simulink subsystem "Transition_Baseline"  (R2024a)
settings: Solver=VariableStepAuto  StartTime=0.0  StopTime=10.0  RelTol=1e-3
undefined symbols (not defined in the file): Kr_transition, Kx_transition, SimIn, SimPar
libraries: simulink_extras x23, ComponentsLib x11, AdaptiveLib x1, libAxisTransformations x1
settings Model: Creator=tbritton  LastModifiedBy=texba
settings SolverCC: AlgebraicLoopSolver=TrustRegion
settings OptimizationCC: ReuseModelBlockBuffer=off
settings DebuggingCC: UnconnectedInputMsg=warning  UnconnectedOutputMsg=warning  UnconnectedLineMsg=warning
settings ModelReferenceCC: EnableRefExpFcnMdlSchedulingChecks=on
settings RTWCC: GPUComputeCapability=3.5  DLArmComputeVersion=19.05

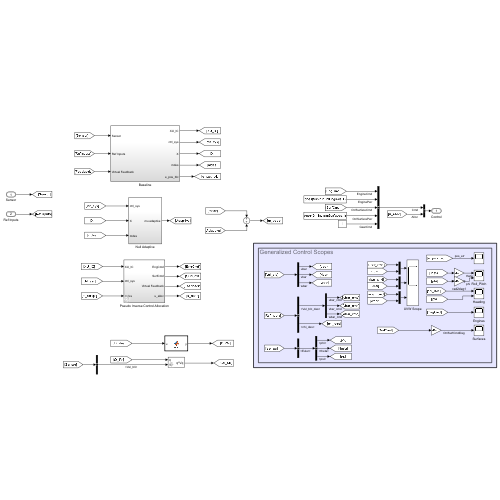
[thumbnail: Simulink's stored preview of the top-level diagram]
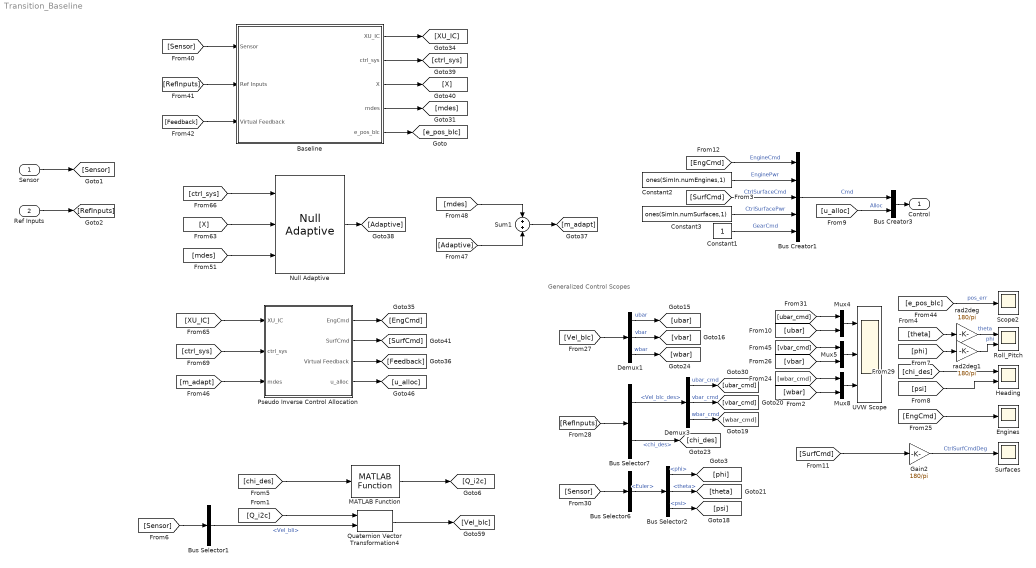
== system Transition_Baseline ==
  note: Generalized Control Scopes
  Sensor : Inport  OutDataTypeStr=Bus: SensorBus
  Ref Inputs : Inport  Port=2  OutDataTypeStr=Bus: BUS_REF_INPUT
  Baseline : Subsystem
      settings: LibrarySourceBlock=ControllersLib/Baseline
  Bus Creator1 : BusCreator  Inputs=5  OutDataTypeStr=Bus: BUS_CMD
  Bus Creator3 : BusCreator  Inputs=2
  Bus Selector1 : BusSelector  OutputSignals=Vel_bIi
  Bus Selector2 : BusSelector  OutputSignals=phi,theta,psi
  Bus Selector6 : BusSelector  OutputSignals=Euler
  Bus Selector7 : BusSelector  OutputSignals=Vel_bIc_des,chi_des
  Constant1 : Constant
  Constant2 : Constant  Value=ones(SimIn.numEngines,1)
  Constant3 : Constant  Value=ones(SimIn.numSurfaces,1)
  Demux1 : Demux  Outputs=3
  Demux3 : Demux  Outputs=3
  Engines : Scope
  Gain2 : Gain  Gain=180/pi
  Heading : Scope  NumInputPorts=2
  MATLAB Function : ComponentsLib/ConvertToControlFrame/MATLAB Function  SystemSampleTime=-1  VariantActivationTime=update diagram  AllowFlexibleInterface=on  Latency=0  AutoFrameSizeCalculation=off
      settings: SourceProductName=Components
  Mux4 : Mux  Inputs=2
  Mux5 : Mux  Inputs=2
  Mux8 : Mux  Inputs=2
  Null Adaptive : AdaptiveLib/Null Adaptive  SystemSampleTime=-1  VariantActivationTime=update diagram  AllowFlexibleInterface=on  Latency=0  AutoFrameSizeCalculation=off
      settings: SourceProductName=Adaptive Augmentation
  Pseudo Inverse Control Allocation : Subsystem  AncestorBlock=AllocatorsLib/Pseudo Inverse Control Allocation
      settings: LibrarySourceBlock=AllocatorsLib/Pseudo Inverse Control Allocation
  Quaternion Vector Transformation4 : libAxisTransformations/Quaternion Vector Transformation  n=0
  Roll_Pitch : Scope  NumInputPorts=2
  Scope2 : Scope
  Sum1 : Sum
  Surfaces : Scope
  UVW Scope : Scope  NumInputPorts=3
  rad2deg : Gain  Gain=180/pi
  rad2deg1 : Gain  Gain=180/pi
  Control : Outport  OutDataTypeStr=Bus: BUS_CONTROL  VectorParamsAs1DForOutWhenUnconnected=off
  wires:
  Baseline/5(e_pos_blc) -> [e_pos_bIc]
  Demux1/1 -> [ubar]  "ubar"
  Mux4/1 -> UVW Scope/1
  Demux3/3 -> [wbar_cmd]  "wbar_cmd"
  Mux5/1 -> UVW Scope/2
  [vbar_cmd] -> Mux5/1
  [ubar_cmd] -> Mux4/1
  [vbar] -> Mux5/2
  [SurfCmd] -> Gain2/1
  [chi_des] -> Heading/1
  [ubar] -> Mux4/2
  [Sensor] -> Bus Selector6/1
  [RefInputs] -> Bus Selector7/1
  [wbar] -> Mux8/2
  [phi] -> rad2deg1/1
  Demux3/2 -> [vbar_cmd]  "vbar_cmd"
  [e_pos_bIc] -> Scope2/1  "pos_err"
  Bus Selector6/1 -> Bus Selector2/1  "<Euler>"
  Bus Selector2/1 -> [phi]  "<phi>"
  Mux8/1 -> UVW Scope/3
  Bus Selector2/3 -> [psi]  "<psi>"
  Gain2/1 -> Surfaces/1  "CtrlSurfCmdDeg"
  [theta] -> rad2deg/1
  Bus Selector2/2 -> [theta]  "<theta>"
  [psi] -> Heading/2
  Demux1/2 -> [vbar]  "vbar"
  [EngCmd] -> Engines/1
  Bus Selector7/1 -> Demux3/1  "<Vel_bIc_des>"
  Demux3/1 -> [ubar_cmd]  "ubar_cmd"
  [Vel_bIc] -> Demux1/1
  Bus Selector7/2 -> [chi_des]  "<chi_des>"
  [wbar_cmd] -> Mux8/1
  Demux1/3 -> [wbar]  "wbar"
  [Sensor] -> Bus Selector1/1
  MATLAB Function/1 -> [Q_i2c]
  Quaternion Vector Transformation4/1 -> [Vel_bIc]
  [chi_des] -> MATLAB Function/1
  [Q_i2c] -> Quaternion Vector Transformation4/1
  Bus Selector1/1 -> Quaternion Vector Transformation4/2  "<Vel_bIi>"
  [ctrl_sys] -> Pseudo Inverse Control Allocation/2(ctrl_sys)
  [XU_IC] -> Pseudo Inverse Control Allocation/1(XU_IC)
  Pseudo Inverse Control Allocation/4(u_alloc) -> [u_alloc]
  Pseudo Inverse Control Allocation/2(SurfCmd) -> [SurfCmd]
  [Adaptive] -> Sum1/2
  [mdes] -> Sum1/1
  Sum1/1 -> [m_adapt]
  Baseline/3(X) -> [X]
  Baseline/2(ctrl_sys) -> [ctrl_sys]
  Null Adaptive/1 -> [Adaptive]
  [X] -> Null Adaptive/2
  [mdes] -> Null Adaptive/3
  [ctrl_sys] -> Null Adaptive/1
  Pseudo Inverse Control Allocation/1(EngCmd) -> [EngCmd]
  Baseline/1(XU_IC) -> [XU_IC]
  Pseudo Inverse Control Allocation/3(Virtual Feedback) -> [Feedback]
  [m_adapt] -> Pseudo Inverse Control Allocation/3(mdes)
  Baseline/4(mdes) -> [mdes]
  [Feedback] -> Baseline/3(Virtual Feedback)
  [RefInputs] -> Baseline/2(Ref Inputs)
  [Sensor] -> Baseline/1(Sensor)
  Constant3/1 -> Bus Creator1/4  "CtrlSurfacePwr"
  Constant2/1 -> Bus Creator1/2  "EnginePwr"
  [EngCmd] -> Bus Creator1/1  "EngineCmd"
  Sensor/1 -> [Sensor]
  Bus Creator1/1 -> Bus Creator3/1  "Cmd"
  [SurfCmd] -> Bus Creator1/3  "CtrlSurfaceCmd"
  Constant1/1 -> Bus Creator1/5  "GearCmd"
  Bus Creator3/1 -> Control/1
  [u_alloc] -> Bus Creator3/2  "Alloc"
  Ref Inputs/1 -> [RefInputs]
  rad2deg/1 -> Roll_Pitch/1  "theta"
  rad2deg1/1 -> Roll_Pitch/2  "phi"

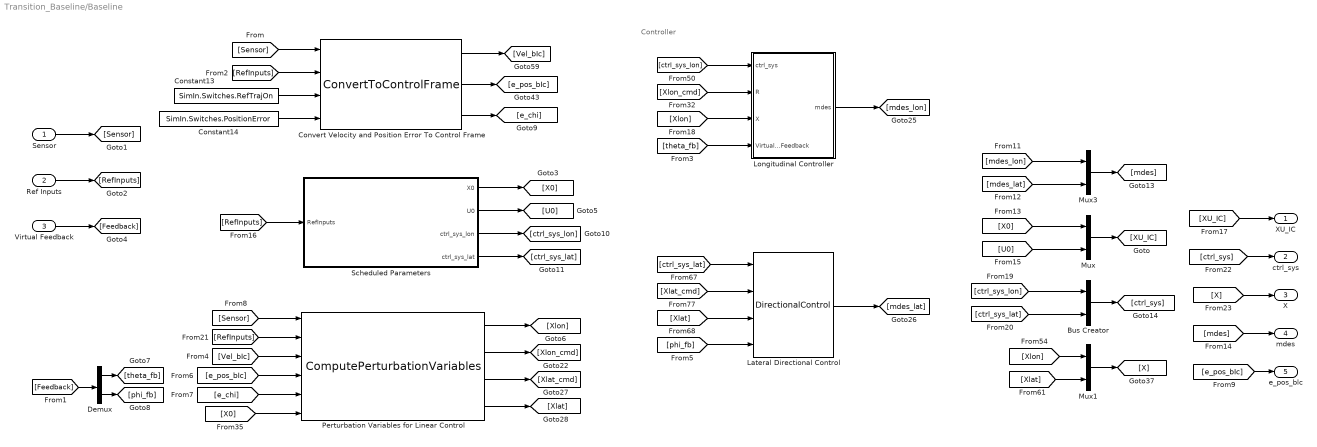
== system Transition_Baseline/Baseline ==
  note: Controller
  Sensor : Inport  OutDataTypeStr=Bus: SensorBus
  Ref Inputs : Inport  Port=2  OutDataTypeStr=Bus: BUS_REF_INPUT
  Virtual Feedback : Inport  Port=3
  Bus Creator : BusCreator  Inputs=2
  Constant13 : Constant  Value=SimIn.Switches.RefTrajOn
  Constant14 : Constant  Value=SimIn.Switches.PositionError
  Convert Velocity and Position Error To Control Frame : ComponentsLib/ConvertToControlFrame  SystemSampleTime=-1  VariantActivationTime=update diagram  AllowFlexibleInterface=on  Latency=0  AutoFrameSizeCalculation=off
      link override delta_cos: Inputs=|++
      settings: SourceProductName=Components
  Demux : Demux  Outputs=2
  Lateral Directional Control : ComponentsLib/DirectionalControl  SystemSampleTime=-1  VariantActivationTime=update diagram  AllowFlexibleInterface=on  Latency=0  AutoFrameSizeCalculation=off
      settings: SourceProductName=Components
  Longitudinal Controller : Subsystem
  Mux : Mux  Inputs=2
  Mux1 : Mux  Inputs=2
  Mux3 : Mux  Inputs=2
  Perturbation Variables for Linear Control : ComponentsLib/ComputePerturbationVariables  SystemSampleTime=-1  VariantActivationTime=update diagram  AllowFlexibleInterface=on  Latency=0  AutoFrameSizeCalculation=off
      settings: SourceProductName=Components
  Scheduled Parameters : Subsystem  AncestorBlock=ComponentsLib/FeedbackScheduling
      settings: LibrarySourceBlock=ComponentsLib/FeedbackScheduling
  XU_IC : Outport
  ctrl_sys : Outport  Port=2
  X : Outport  Port=3
  mdes : Outport  Port=4
  e_pos_blc : Outport  Port=5
  wires:
  [X] -> X/1
  [Xlat] -> Mux1/2
  [Xlon] -> Mux1/1
  Mux1/1 -> [X]
  [ctrl_sys] -> ctrl_sys/1
  Bus Creator/1 -> [ctrl_sys]
  [ctrl_sys_lat] -> Bus Creator/2
  [ctrl_sys_lon] -> Bus Creator/1
  [XU_IC] -> XU_IC/1
  Mux/1 -> [XU_IC]
  [U0] -> Mux/2
  [X0] -> Mux/1
  [mdes] -> mdes/1
  Mux3/1 -> [mdes]
  [mdes_lon] -> Mux3/1
  [phi_fb] -> Lateral Directional Control/4
  [theta_fb] -> Longitudinal Controller/4(Virtual Feedback)
  Demux/1 -> [theta_fb]
  Demux/2 -> [phi_fb]
  [Feedback] -> Demux/1
  Virtual Feedback/1 -> [Feedback]
  [Xlat_cmd] -> Lateral Directional Control/2
  [Xlon] -> Longitudinal Controller/3(X)
  [Xlat] -> Lateral Directional Control/3
  Longitudinal Controller/1(mdes) -> [mdes_lon]
  [ctrl_sys_lon] -> Longitudinal Controller/1(ctrl_sys)
  [ctrl_sys_lat] -> Lateral Directional Control/1
  Lateral Directional Control/1 -> [mdes_lat]
  [Xlon_cmd] -> Longitudinal Controller/2(R)
  Scheduled Parameters/4(ctrl_sys_lat) -> [ctrl_sys_lat]
  Scheduled Parameters/2(U0) -> [U0]
  [e_chi] -> Perturbation Variables for Linear Control/5
  Constant14/1 -> Convert Velocity and Position Error To Control Frame/4
  [RefInputs] -> Perturbation Variables for Linear Control/2
  Constant13/1 -> Convert Velocity and Position Error To Control Frame/3
  [Vel_bIc] -> Perturbation Variables for Linear Control/3
  [Sensor] -> Convert Velocity and Position Error To Control Frame/1
  Convert Velocity and Position Error To Control Frame/3 -> [e_chi]
  Perturbation Variables for Linear Control/2 -> [Xlon_cmd]
  [RefInputs] -> Scheduled Parameters/1(RefInputs)
  Perturbation Variables for Linear Control/4 -> [Xlat]
  [e_pos_bIc] -> Perturbation Variables for Linear Control/4
  Scheduled Parameters/3(ctrl_sys_lon) -> [ctrl_sys_lon]
  Convert Velocity and Position Error To Control Frame/2 -> [e_pos_bIc]
  Convert Velocity and Position Error To Control Frame/1 -> [Vel_bIc]
  [RefInputs] -> Convert Velocity and Position Error To Control Frame/2
  Ref Inputs/1 -> [RefInputs]
  Scheduled Parameters/1(X0) -> [X0]
  Sensor/1 -> [Sensor]
  Perturbation Variables for Linear Control/3 -> [Xlat_cmd]
  [Sensor] -> Perturbation Variables for Linear Control/1
  Perturbation Variables for Linear Control/1 -> [Xlon]
  [X0] -> Perturbation Variables for Linear Control/6
  [e_pos_bIc] -> e_pos_blc/1
  [mdes_lat] -> Mux3/2

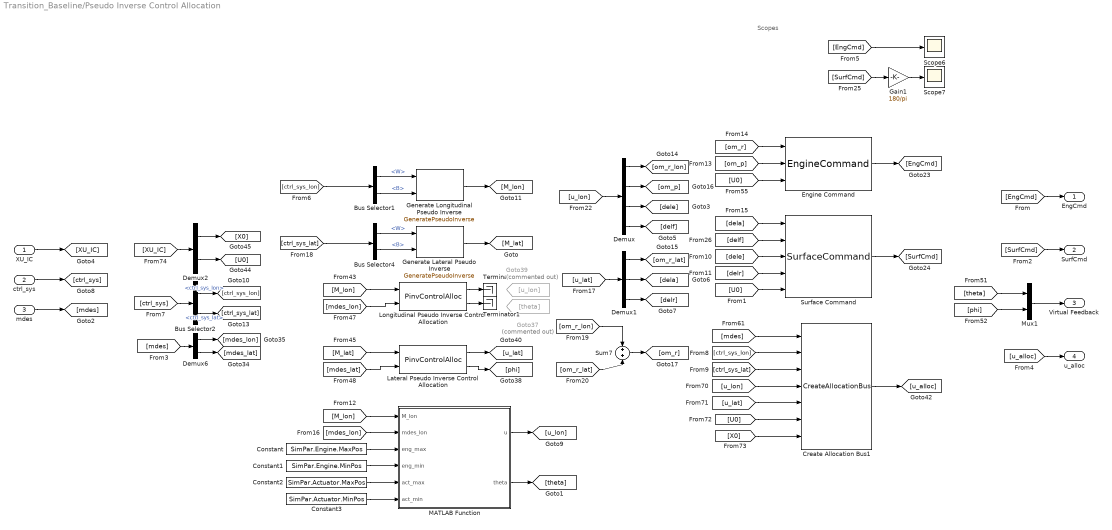
== system Transition_Baseline/Pseudo Inverse Control Allocation ==
  note: Scopes
  XU_IC : Inport
  ctrl_sys : Inport  Port=2
  mdes : Inport  Port=3
  Bus Selector1 : BusSelector  OutputSignals=W,B
  Bus Selector2 : BusSelector  OutputSignals=ctrl_sys_lon,ctrl_sys_lat
  Bus Selector4 : BusSelector  OutputSignals=W,B
  Constant : Constant  Value=SimPar.Engine.MaxPos
  Constant1 : Constant  Value=SimPar.Engine.MinPos
  Constant2 : Constant  Value=SimPar.Actuator.MaxPos
  Constant3 : Constant  Value=SimPar.Actuator.MinPos
  Create Allocation Bus1 : ComponentsLib/CreateAllocationBus  SystemSampleTime=-1  VariantActivationTime=update diagram  AllowFlexibleInterface=on  Latency=0  AutoFrameSizeCalculation=off
      settings: SourceProductName=Components
  Demux : Demux  Outputs=[8 1 1 1]
  Demux1 : Demux  Outputs=[8 1 1]
  Demux2 : Demux  Outputs=[12 13]
  Demux6 : Demux  Outputs=[3 3]
  Engine Command : ComponentsLib/EngineCommand  SystemSampleTime=-1  VariantActivationTime=update diagram  AllowFlexibleInterface=on  Latency=0  AutoFrameSizeCalculation=off
      settings: SourceProductName=Components
  Gain1 : Gain  Gain=180/pi
  Generate Lateral Pseudo Inverse : ComponentsLib/GeneratePseudoInverse  SystemSampleTime=-1  VariantActivationTime=update diagram  AllowFlexibleInterface=on  Latency=0  AutoFrameSizeCalculation=off
      settings: SourceProductName=Components
  Generate Longitudinal Pseudo Inverse : ComponentsLib/GeneratePseudoInverse  SystemSampleTime=-1  VariantActivationTime=update diagram  AllowFlexibleInterface=on  Latency=0  AutoFrameSizeCalculation=off
      settings: SourceProductName=Components
  Goto37 : Goto  Commented=on  GotoTag=theta
  Goto39 : Goto  Commented=on  GotoTag=u_lon
  Lateral Pseudo Inverse Control Allocation : ComponentsLib/PinvControlAlloc  SystemSampleTime=-1  VariantActivationTime=update diagram  AllowFlexibleInterface=on  Latency=0  AutoFrameSizeCalculation=off
      settings: SourceProductName=Components
  Longitudinal Pseudo Inverse Control Allocation : ComponentsLib/PinvControlAlloc  SystemSampleTime=-1  VariantActivationTime=update diagram  AllowFlexibleInterface=on  Latency=0  AutoFrameSizeCalculation=off
      settings: SourceProductName=Components
  MATLAB Function : MATLAB Function  TreatAsAtomicUnit=on
  Mux1 : Mux  Inputs=2
  Scope6 : Scope
  Scope7 : Scope
  Sum7 : Sum
  Surface Command : ComponentsLib/SurfaceCommand  SystemSampleTime=-1  VariantActivationTime=update diagram  AllowFlexibleInterface=on  Latency=0  AutoFrameSizeCalculation=off
      settings: SourceProductName=Components
  Terminator : Terminator
  Terminator1 : Terminator
  EngCmd : Outport
  SurfCmd : Outport  Port=2
  Virtual Feedback : Outport  Port=3
  u_alloc : Outport  Port=4
  wires:
  Constant/1 -> MATLAB Function/3(eng_max)
  Constant1/1 -> MATLAB Function/4(eng_min)
  Constant2/1 -> MATLAB Function/5(act_max)
  Constant3/1 -> MATLAB Function/6(act_min)
  MATLAB Function/2(theta) -> [theta]
  MATLAB Function/1(u) -> [u_lon]
  [mdes_lon] -> MATLAB Function/2(mdes_lon)
  [M_lon] -> MATLAB Function/1(M_lon)
  [ctrl_sys_lat] -> Create Allocation Bus1/3
  [ctrl_sys_lon] -> Create Allocation Bus1/2
  Bus Selector2/2 -> [ctrl_sys_lat]  "<ctrl_sys_lat>"
  Bus Selector2/1 -> [ctrl_sys_lon]  "<ctrl_sys_lon>"
  [ctrl_sys] -> Bus Selector2/1
  Bus Selector1/2 -> Generate Longitudinal Pseudo Inverse/2  "<B>"
  Bus Selector4/2 -> Generate Lateral Pseudo Inverse/2  "<B>"
  Generate Lateral Pseudo Inverse/1 -> [M_lat]
  Bus Selector4/1 -> Generate Lateral Pseudo Inverse/1  "<W>"
  Generate Longitudinal Pseudo Inverse/1 -> [M_lon]
  [ctrl_sys_lon] -> Bus Selector1/1
  Bus Selector1/1 -> Generate Longitudinal Pseudo Inverse/1  "<W>"
  [ctrl_sys_lat] -> Bus Selector4/1
  [EngCmd] -> Scope6/1
  [SurfCmd] -> Gain1/1
  Gain1/1 -> Scope7/1
  [u_alloc] -> u_alloc/1
  ctrl_sys/1 -> [ctrl_sys]
  XU_IC/1 -> [XU_IC]
  mdes/1 -> [mdes]
  [mdes] -> Demux6/1
  Demux6/1 -> [mdes_lon]
  Demux6/2 -> [mdes_lat]
  [mdes] -> Create Allocation Bus1/1
  Demux2/1 -> [X0]
  [X0] -> Create Allocation Bus1/7
  [XU_IC] -> Demux2/1
  [u_lat] -> Create Allocation Bus1/5
  Create Allocation Bus1/1 -> [u_alloc]
  [u_lon] -> Create Allocation Bus1/4
  [U0] -> Create Allocation Bus1/6
  Demux2/2 -> [U0]
  [SurfCmd] -> SurfCmd/1
  [EngCmd] -> EngCmd/1
  [dela] -> Surface Command/1
  [U0] -> Surface Command/5
  [om_r] -> Engine Command/1
  [om_p] -> Engine Command/2
  [delr] -> Surface Command/4
  [delf] -> Surface Command/2
  [dele] -> Surface Command/3
  [U0] -> Engine Command/3
  Surface Command/1 -> [SurfCmd]
  Engine Command/1 -> [EngCmd]
  Demux1/3 -> [delr]
  Demux/4 -> [delf]
  Demux/1 -> [om_r_lon]
  Demux1/1 -> [om_r_lat]
  Demux1/2 -> [dela]
  [u_lon] -> Demux/1
  Sum7/1 -> [om_r]
  [om_r_lon] -> Sum7/1
  [om_r_lat] -> Sum7/2
  [u_lat] -> Demux1/1
  Demux/2 -> [om_p]
  Demux/3 -> [dele]
  [M_lat] -> Lateral Pseudo Inverse Control Allocation/1
  [M_lon] -> Longitudinal Pseudo Inverse Control Allocation/1
  Mux1/1 -> Virtual Feedback/1
  Longitudinal Pseudo Inverse Control Allocation/2 -> Terminator1/1
  Lateral Pseudo Inverse Control Allocation/1 -> [u_lat]
  [mdes_lon] -> Longitudinal Pseudo Inverse Control Allocation/2
  [phi] -> Mux1/2
  [mdes_lat] -> Lateral Pseudo Inverse Control Allocation/2
  [theta] -> Mux1/1
  Longitudinal Pseudo Inverse Control Allocation/1 -> Terminator/1
  Lateral Pseudo Inverse Control Allocation/2 -> [phi]

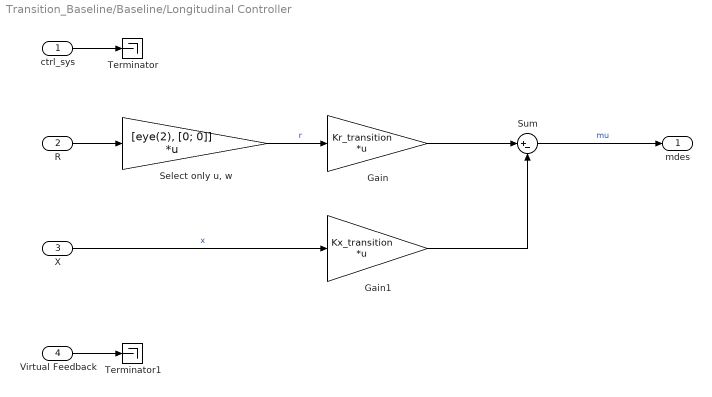
== system Transition_Baseline/Baseline/Longitudinal Controller ==
  ctrl_sys : Inport
  R : Inport  Port=2
  X : Inport  Port=3
  Virtual Feedback : Inport  Port=4
  Gain : Gain  Gain=Kr_transition  Multiplication=Matrix(K*u)
  Gain1 : Gain  Gain=Kx_transition  Multiplication=Matrix(K*u)
  "Select only u, w" : Gain  Gain=[eye(2), [0; 0]]  Multiplication=Matrix(K*u)
  Sum : Sum  Inputs=|+-
  Terminator : Terminator
  Terminator1 : Terminator
  mdes : Outport
  wires:
  ctrl_sys/1 -> Terminator/1
  Virtual Feedback/1 -> Terminator1/1
  R/1 -> "Select only u, w"/1
  "Select only u, w"/1 -> Gain/1  "r"
  Gain/1 -> Sum/1
  X/1 -> Gain1/1  "x"
  Gain1/1 -> Sum/2
  Sum/1 -> mdes/1  "mu"

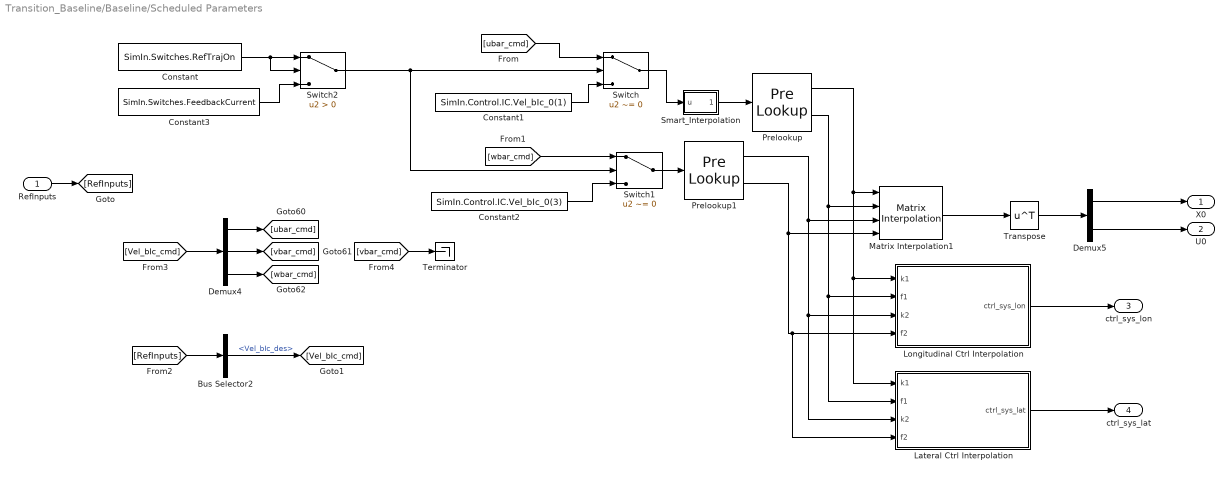
== system Transition_Baseline/Baseline/Scheduled Parameters ==
  RefInputs : Inport  OutDataTypeStr=Bus: BUS_REF_INPUT
  Bus Selector2 : BusSelector  OutputSignals=Vel_bIc_des
  Constant : Constant  Value=SimIn.Switches.RefTrajOn
  Constant1 : Constant  Value=SimIn.Control.IC.Vel_bIc_0(1)
  Constant2 : Constant  Value=SimIn.Control.IC.Vel_bIc_0(3)
  Constant3 : Constant  Value=SimIn.Switches.FeedbackCurrent
  Demux4 : Demux  Outputs=3
  Demux5 : Demux  Outputs=[12 13]
  Lateral Ctrl Interpolation : Subsystem
  Longitudinal Ctrl Interpolation : Subsystem
  Matrix Interpolation1 : simulink_extras/Additional Lookup Tables/Matrix Interpolation  InterpMethod=Linear  ExtrapMethod=Clip  InterpolateDimension=2  TableData=SimIn.Control.trim.XU0_interp  SimulateUsing=Code generation
  Prelookup : PreLookup  BreakpointsData=SimIn.Control.trim.UH
  Prelookup1 : PreLookup  BreakpointsData=SimIn.Control.trim.WH
  Smart_Interpolation : MATLAB Function  TreatAsAtomicUnit=on
  Switch : Switch  Criteria=u2 ~= 0  SaturateOnIntegerOverflow=off  InputSameDT=off
  Switch1 : Switch  Criteria=u2 ~= 0  SaturateOnIntegerOverflow=off  InputSameDT=off
  Switch2 : Switch  Criteria=u2 > Threshold  SaturateOnIntegerOverflow=off  InputSameDT=off
  Terminator : Terminator
  Transpose : Math  Operator=transpose
  X0 : Outport
  U0 : Outport  Port=2
  ctrl_sys_lon : Outport  Port=3
  ctrl_sys_lat : Outport  Port=4
  wires:
  [wbar_cmd] -> Switch1/1
  [vbar_cmd] -> Terminator/1
  Bus Selector2/1 -> [Vel_bIc_cmd]  "<Vel_bIc_des>"
  [RefInputs] -> Bus Selector2/1
  [ubar_cmd] -> Switch/1
  RefInputs/1 -> [RefInputs]
  [Vel_bIc_cmd] -> Demux4/1
  Demux4/2 -> [vbar_cmd]
  Demux4/3 -> [wbar_cmd]
  Demux4/1 -> [ubar_cmd]
  Matrix Interpolation1/1 -> Transpose/1
  Transpose/1 -> Demux5/1
  Demux5/1 -> X0/1
  Demux5/2 -> U0/1
  Prelookup1/1 -> Longitudinal Ctrl Interpolation/3(k2), Lateral Ctrl Interpolation/3(k2), Matrix Interpolation1/3
  Prelookup1/2 -> Longitudinal Ctrl Interpolation/4(f2), Lateral Ctrl Interpolation/4(f2), Matrix Interpolation1/4
  Lateral Ctrl Interpolation/1(ctrl_sys_lat) -> ctrl_sys_lat/1
  Longitudinal Ctrl Interpolation/1(ctrl_sys_lon) -> ctrl_sys_lon/1
  Constant1/1 -> Switch/3
  Switch1/1 -> Prelookup1/1
  Constant2/1 -> Switch1/3
  Switch2/1 -> Switch1/2, Switch/2
  Constant/1 -> Switch2/1, Switch2/2
  Constant3/1 -> Switch2/3
  Switch/1 -> Smart_Interpolation/1(u)
  Smart_Interpolation/1(u_out) -> Prelookup/1
  Prelookup/2 -> Longitudinal Ctrl Interpolation/2(f1), Lateral Ctrl Interpolation/2(f1), Matrix Interpolation1/2
  Prelookup/1 -> Matrix Interpolation1/1, Longitudinal Ctrl Interpolation/1(k1), Lateral Ctrl Interpolation/1(k1)

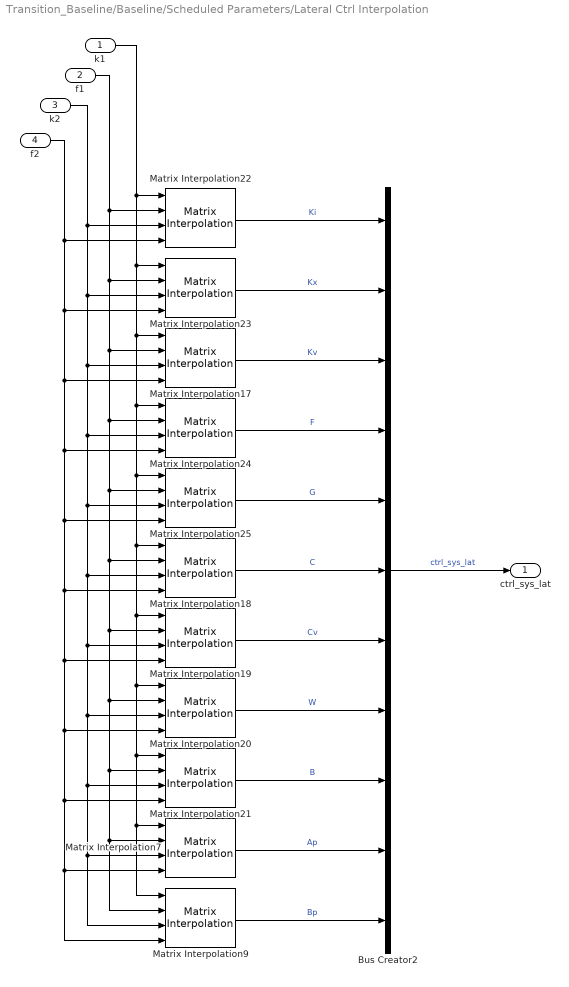
== system Transition_Baseline/Baseline/Scheduled Parameters/Lateral Ctrl Interpolation ==
  k1 : Inport
  f1 : Inport  Port=2
  k2 : Inport  Port=3
  f2 : Inport  Port=4
  Bus Creator2 : BusCreator  Inputs=11
  Matrix Interpolation17 : simulink_extras/Additional Lookup Tables/Matrix Interpolation  InterpMethod=Linear  ExtrapMethod=Clip  InterpolateDimension=2  TableData=SimIn.Control.trim.Kv_lat_interp  SimulateUsing=Code generation
  Matrix Interpolation18 : simulink_extras/Additional Lookup Tables/Matrix Interpolation  InterpMethod=Linear  ExtrapMethod=Clip  InterpolateDimension=2  TableData=SimIn.Control.trim.C_lat_interp  SimulateUsing=Code generation
  Matrix Interpolation19 : simulink_extras/Additional Lookup Tables/Matrix Interpolation  InterpMethod=Linear  ExtrapMethod=Clip  InterpolateDimension=2  TableData=SimIn.Control.trim.Cv_lat_interp  SimulateUsing=Code generation
  Matrix Interpolation20 : simulink_extras/Additional Lookup Tables/Matrix Interpolation  InterpMethod=Linear  ExtrapMethod=Clip  InterpolateDimension=2  TableData=SimIn.Control.trim.W_lat_interp  SimulateUsing=Code generation
  Matrix Interpolation21 : simulink_extras/Additional Lookup Tables/Matrix Interpolation  InterpMethod=Linear  ExtrapMethod=Clip  InterpolateDimension=2  TableData=SimIn.Control.trim.B_lat_interp  SimulateUsing=Code generation
  Matrix Interpolation22 : simulink_extras/Additional Lookup Tables/Matrix Interpolation  InterpMethod=Linear  ExtrapMethod=Clip  InterpolateDimension=2  TableData=SimIn.Control.trim.Ki_lat_interp  SimulateUsing=Code generation
  Matrix Interpolation23 : simulink_extras/Additional Lookup Tables/Matrix Interpolation  InterpMethod=Linear  ExtrapMethod=Clip  InterpolateDimension=2  TableData=SimIn.Control.trim.Kx_lat_interp  SimulateUsing=Code generation
  Matrix Interpolation24 : simulink_extras/Additional Lookup Tables/Matrix Interpolation  InterpMethod=Linear  ExtrapMethod=Clip  InterpolateDimension=2  TableData=SimIn.Control.trim.F_lat_interp  SimulateUsing=Code generation
  Matrix Interpolation25 : simulink_extras/Additional Lookup Tables/Matrix Interpolation  InterpMethod=Linear  ExtrapMethod=Clip  InterpolateDimension=2  TableData=SimIn.Control.trim.G_lat_interp  SimulateUsing=Code generation
  Matrix Interpolation7 : simulink_extras/Additional Lookup Tables/Matrix Interpolation  InterpMethod=Linear  ExtrapMethod=Clip  InterpolateDimension=2  TableData=SimIn.Control.trim.Ap_lat_interp  SimulateUsing=Code generation
  Matrix Interpolation9 : simulink_extras/Additional Lookup Tables/Matrix Interpolation  InterpMethod=Linear  ExtrapMethod=Clip  InterpolateDimension=2  TableData=SimIn.Control.trim.Bp_lat_interp  SimulateUsing=Code generation
  ctrl_sys_lat : Outport
  wires:
  k1/1 -> Matrix Interpolation22/1, Matrix Interpolation23/1, Matrix Interpolation17/1, Matrix Interpolation25/1, Matrix Interpolation18/1, Matrix Interpolation19/1, Matrix Interpolation21/1, Matrix Interpolation9/1, Matrix Interpolation7/1, Matrix Interpolation20/1, Matrix Interpolation24/1
  k2/1 -> Matrix Interpolation22/3, Matrix Interpolation23/3, Matrix Interpolation17/3, Matrix Interpolation24/3, Matrix Interpolation25/3, Matrix Interpolation18/3, Matrix Interpolation19/3, Matrix Interpolation20/3, Matrix Interpolation21/3, Matrix Interpolation7/3, Matrix Interpolation9/3
  Matrix Interpolation20/1 -> Bus Creator2/8  "W"
  f2/1 -> Matrix Interpolation22/4, Matrix Interpolation23/4, Matrix Interpolation17/4, Matrix Interpolation24/4, Matrix Interpolation25/4, Matrix Interpolation18/4, Matrix Interpolation19/4, Matrix Interpolation20/4, Matrix Interpolation21/4, Matrix Interpolation7/4, Matrix Interpolation9/4
  f1/1 -> Matrix Interpolation22/2, Matrix Interpolation23/2, Matrix Interpolation17/2, Matrix Interpolation24/2, Matrix Interpolation25/2, Matrix Interpolation18/2, Matrix Interpolation19/2, Matrix Interpolation20/2, Matrix Interpolation21/2, Matrix Interpolation7/2, Matrix Interpolation9/2
  Matrix Interpolation22/1 -> Bus Creator2/1  "Ki"
  Matrix Interpolation17/1 -> Bus Creator2/3  "Kv"
  Matrix Interpolation18/1 -> Bus Creator2/6  "C"
  Matrix Interpolation19/1 -> Bus Creator2/7  "Cv"
  Matrix Interpolation23/1 -> Bus Creator2/2  "Kx"
  Matrix Interpolation9/1 -> Bus Creator2/11  "Bp"
  Matrix Interpolation25/1 -> Bus Creator2/5  "G"
  Matrix Interpolation24/1 -> Bus Creator2/4  "F"
  Matrix Interpolation21/1 -> Bus Creator2/9  "B"
  Matrix Interpolation7/1 -> Bus Creator2/10  "Ap"
  Bus Creator2/1 -> ctrl_sys_lat/1  "ctrl_sys_lat"

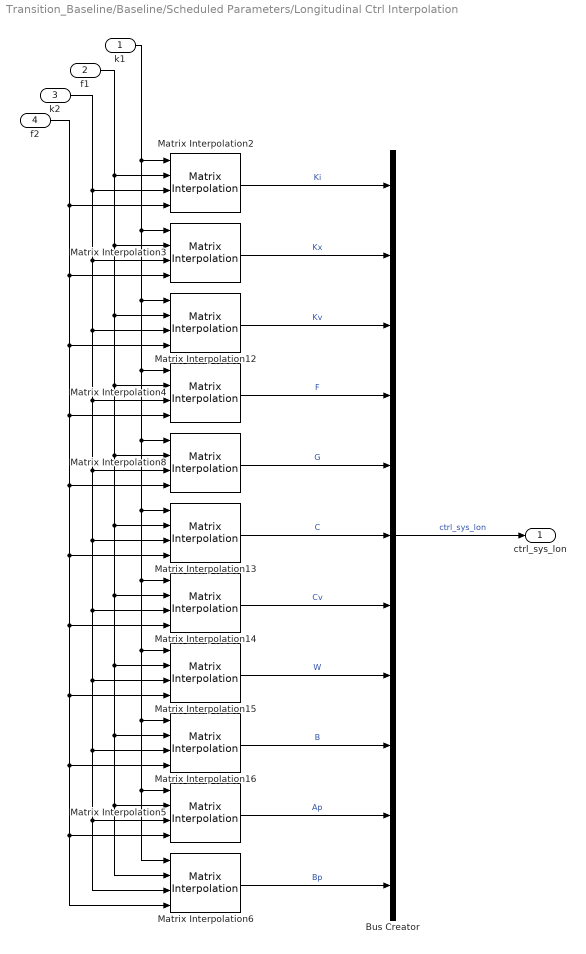
== system Transition_Baseline/Baseline/Scheduled Parameters/Longitudinal Ctrl Interpolation ==
  k1 : Inport
  f1 : Inport  Port=2
  k2 : Inport  Port=3
  f2 : Inport  Port=4
  Bus Creator : BusCreator  Inputs=11
  Matrix Interpolation12 : simulink_extras/Additional Lookup Tables/Matrix Interpolation  InterpMethod=Linear  ExtrapMethod=Clip  InterpolateDimension=2  TableData=SimIn.Control.trim.Kv_lon_interp  SimulateUsing=Code generation
  Matrix Interpolation13 : simulink_extras/Additional Lookup Tables/Matrix Interpolation  InterpMethod=Linear  ExtrapMethod=Clip  InterpolateDimension=2  TableData=SimIn.Control.trim.C_lon_interp  SimulateUsing=Code generation
  Matrix Interpolation14 : simulink_extras/Additional Lookup Tables/Matrix Interpolation  InterpMethod=Linear  ExtrapMethod=Clip  InterpolateDimension=2  TableData=SimIn.Control.trim.Cv_lon_interp  SimulateUsing=Code generation
  Matrix Interpolation15 : simulink_extras/Additional Lookup Tables/Matrix Interpolation  InterpMethod=Linear  ExtrapMethod=Clip  InterpolateDimension=2  TableData=SimIn.Control.trim.W_lon_interp  SimulateUsing=Code generation
  Matrix Interpolation16 : simulink_extras/Additional Lookup Tables/Matrix Interpolation  InterpMethod=Linear  ExtrapMethod=Clip  InterpolateDimension=2  TableData=SimIn.Control.trim.B_lon_interp  SimulateUsing=Code generation
  Matrix Interpolation2 : simulink_extras/Additional Lookup Tables/Matrix Interpolation  InterpMethod=Linear  ExtrapMethod=Clip  InterpolateDimension=2  TableData=SimIn.Control.trim.Ki_lon_interp  SimulateUsing=Code generation
  Matrix Interpolation3 : simulink_extras/Additional Lookup Tables/Matrix Interpolation  InterpMethod=Linear  ExtrapMethod=Clip  InterpolateDimension=2  TableData=SimIn.Control.trim.Kx_lon_interp  SimulateUsing=Code generation
  Matrix Interpolation4 : simulink_extras/Additional Lookup Tables/Matrix Interpolation  InterpMethod=Linear  ExtrapMethod=Clip  InterpolateDimension=2  TableData=SimIn.Control.trim.F_lon_interp  SimulateUsing=Code generation
  Matrix Interpolation5 : simulink_extras/Additional Lookup Tables/Matrix Interpolation  InterpMethod=Linear  ExtrapMethod=Clip  InterpolateDimension=2  TableData=SimIn.Control.trim.Ap_lon_interp  SimulateUsing=Code generation
  Matrix Interpolation6 : simulink_extras/Additional Lookup Tables/Matrix Interpolation  InterpMethod=Linear  ExtrapMethod=Clip  InterpolateDimension=2  TableData=SimIn.Control.trim.Bp_lon_interp  SimulateUsing=Code generation
  Matrix Interpolation8 : simulink_extras/Additional Lookup Tables/Matrix Interpolation  InterpMethod=Linear  ExtrapMethod=Clip  InterpolateDimension=2  TableData=SimIn.Control.trim.G_lon_interp  SimulateUsing=Code generation
  ctrl_sys_lon : Outport
  wires:
  f1/1 -> Matrix Interpolation2/2, Matrix Interpolation3/2, Matrix Interpolation12/2, Matrix Interpolation4/2, Matrix Interpolation8/2, Matrix Interpolation13/2, Matrix Interpolation14/2, Matrix Interpolation15/2, Matrix Interpolation16/2, Matrix Interpolation5/2, Matrix Interpolation6/2
  Matrix Interpolation6/1 -> Bus Creator/11  "Bp"
  k2/1 -> Matrix Interpolation2/3, Matrix Interpolation3/3, Matrix Interpolation12/3, Matrix Interpolation4/3, Matrix Interpolation8/3, Matrix Interpolation13/3, Matrix Interpolation14/3, Matrix Interpolation15/3, Matrix Interpolation16/3, Matrix Interpolation5/3, Matrix Interpolation6/3
  k1/1 -> Matrix Interpolation2/1, Matrix Interpolation3/1, Matrix Interpolation12/1, Matrix Interpolation4/1, Matrix Interpolation8/1, Matrix Interpolation13/1, Matrix Interpolation14/1, Matrix Interpolation15/1, Matrix Interpolation5/1, Matrix Interpolation6/1, Matrix Interpolation16/1
  Matrix Interpolation3/1 -> Bus Creator/2  "Kx"
  Matrix Interpolation13/1 -> Bus Creator/6  "C"
  Matrix Interpolation8/1 -> Bus Creator/5  "G"
  Matrix Interpolation16/1 -> Bus Creator/9  "B"
  Matrix Interpolation2/1 -> Bus Creator/1  "Ki"
  Matrix Interpolation14/1 -> Bus Creator/7  "Cv"
  Matrix Interpolation4/1 -> Bus Creator/4  "F"
  Matrix Interpolation5/1 -> Bus Creator/10  "Ap"
  Matrix Interpolation15/1 -> Bus Creator/8  "W"
  Matrix Interpolation12/1 -> Bus Creator/3  "Kv"
  Bus Creator/1 -> ctrl_sys_lon/1  "ctrl_sys_lon"
  f2/1 -> Matrix Interpolation2/4, Matrix Interpolation3/4, Matrix Interpolation12/4, Matrix Interpolation4/4, Matrix Interpolation8/4, Matrix Interpolation13/4, Matrix Interpolation14/4, Matrix Interpolation15/4, Matrix Interpolation16/4, Matrix Interpolation5/4, Matrix Interpolation6/4

== matlab function Transition_Baseline/Baseline/Scheduled Parameters/Smart_Interpolation ==
  data: u input; u_out output
function u_out = fcn(u)

% This function is used to limit interpolation for three portions of the
% flight envelope: 1) Below zero knots, 2) After the end of transition
% (90 kts) and before cruise (100 knots) and 3) above the last trim map
% point (130 knots)

ft2kts = 0.3048/1852.0*3600; % Conversion factor of ft/sec to knots (derived from setUnits values)
kts2ft = 1/ft2kts; % Conversion factor from knots to ft/sec
if u < 0* kts2ft; % SimIn.Control.trim.UH(1)
    u_out = 0*kts2ft; % SimIn.Control.trim.UH(1);
% elseif u>90*kts2ft && u<100*kts2ft
%     u_out = 100*kts2ft;
elseif u>130*kts2ft % SimIn.Control.trim.UH(end)
    u_out = 130*kts2ft; % SimIn.Control.trim.UH(end)
else
    u_out = u;
end

== matlab function Transition_Baseline/Pseudo Inverse Control Allocation/MATLAB Function ==
  data: M_lon input; u output; mdes_lon input; theta output; eng_max input; eng_min input; act_max input; act_min input
function [u, theta] = Limited_Allocation(M_lon, mdes_lon, eng_max, eng_min, act_max, act_min)

[u, theta] = Limited_Long_Cont_Alloc(M_lon, mdes_lon, eng_max, eng_min, act_max, act_min);
